simulink model "ThrdRwLtStBkReclnTrgtPosSelc"  (R2018b)
settings: Solver=FixedStepDiscrete  StartTime=0.0  StopTime=10.0  FixedStep=0.01  RelTol=1e-3
undefined symbols (not defined in the file or in its folder): KeSMSw6sAcsEntryThdRwLtStBkReclnUpwdDnwdPos_Val, KeSMSw6sAcsEntryThdRwLtStBkReclnUpwdDnwdPosMax_Val, KeSMSw6sAcsEntryThdRwLtStBkReclnUpwdDnwdPosMin_Val, KeSMSw6sLugThdRwLtStBkReclnUpwdDnwdPos_Val, KeSMSw6sLugThdRwLtStBkReclnUpwdDnwdPosMax_Val, KeSMSw6sLugThdRwLtStBkReclnUpwdDnwdPosMin_Val, KeSMSw6sVIPThdRwLtStBkReclnUpwdDnwdPos_Val, KeSMSw6sVIPThdRwLtStBkReclnUpwdDnwdPosMax_Val, KeSMSw6sVIPThdRwLtStBkReclnUpwdDnwdPosMin_Val, KeSMSwAcsEntryThdRwLtStBkReclnUpwdDnwdPos_Val, KeSMSwAcsEntryThdRwLtStBkReclnUpwdDnwdPosMax_Val, KeSMSwAcsEntryThdRwLtStBkReclnUpwdDnwdPosMin_Val, KeSMSwLugThdRwLtStBkReclnUpwdDnwdPos_Val, KeSMSwLugThdRwLtStBkReclnUpwdDnwdPosMax_Val, KeSMSwLugThdRwLtStBkReclnUpwdDnwdPosMin_Val, KeSMSwVIPThdRwLtStBkReclnUpwdDnwdPos_Val, KeSMSwVIPThdRwLtStBkReclnUpwdDnwdPosMax_Val, KeSMSwVIPThdRwLtStBkReclnUpwdDnwdPosMin_Val
libraries: TrgtPosSelcLib x4
settings Model: Creator=sn2xws  LastModifiedBy=sn2xws
settings DataIOCC: SaveFormat=StructureWithTime
settings OptimizationCC: DefaultParameterBehavior=Inlined  EnhancedBackFolding=on  PassReuseOutputArgsAs=Individual arguments  ZeroExternalMemoryAtStartup=off  ZeroInternalMemoryAtStartup=off  OptimizeBlockOrder=speed  DifferentSizesBufferReuse=on  OptimizationCustomize=off
settings DebuggingCC: ParameterTunabilityLossMsg=error
settings ModelReferenceCC: ModelReferenceNumInstancesAllowed=Single
settings SFSimCC: MATLABDynamicMemAlloc=off
settings RTWCC: SystemTargetFile=autosar.tlc  GenCodeOnly=on  TemplateMakefile=ert_default_tmf  Description=AUTOSAR  GenerateReport=on  IncludeHyperlinkInReport=on  LaunchReport=on  GenerateTraceInfo=on  GenerateTraceReport=on  GenerateTraceReportSl=on  GenerateTraceReportSf=on  GenerateTraceReportEml=on
settings CodeAppCC: ForceParamTrailComments=on  IgnoreCustomStorageClasses=off  OperatorAnnotations=on  SimulinkDataObjDesc=on  SFDataObjDesc=on  InsertBlockDesc=on
settings STFCustomTargetCC: TargetLangStandard=C99 (ISO)  MultiwordLength=256  ParMdlRefBuildCompliant=on  CompOptLevelCompliant=on  IncludeMdlTerminateFcn=off  CombineOutputUpdateFcns=on  SuppressErrorStatus=on  ERTCustomFileBanners=on  SupportNonFinite=off  SupportComplex=off  SupportContinuousTime=off  SupportNonInlinedSFcns=off  RemoveResetFunc=on  MATLABClassNameForMDSCustomization=Simulink.SoftwareTarget.ERTCustomization  AutosarCompliant=on  UseToolchainInfoCompliant=on  LookupTableObjectStructAxisOrder=2,1,3,4,...  LUTObjectStructOrderEvenSpacing=Size,Table,Breakpoints  SystemTargetFile=autosar.tlc
settings ERTTargetCC: TargetLangStandard=C99 (ISO)  ConcurrentExecutionCompliant=off  IncludeMdlTerminateFcn=off  SuppressErrorStatus=on  SupportNonFinite=off  SupportComplex=off  ModelStepFunctionPrototypeControlCompliant=off  CPPClassGenCompliant=off  AutosarCompliant=on  LookupTableObjectStructAxisOrder=2,1,3,4,...  LUTObjectStructOrderEvenSpacing=Size,Table,Breakpoints  InlinedParameterPlacement=NonHierarchical  ERTCustomFileTemplate=example_file_process.tlc

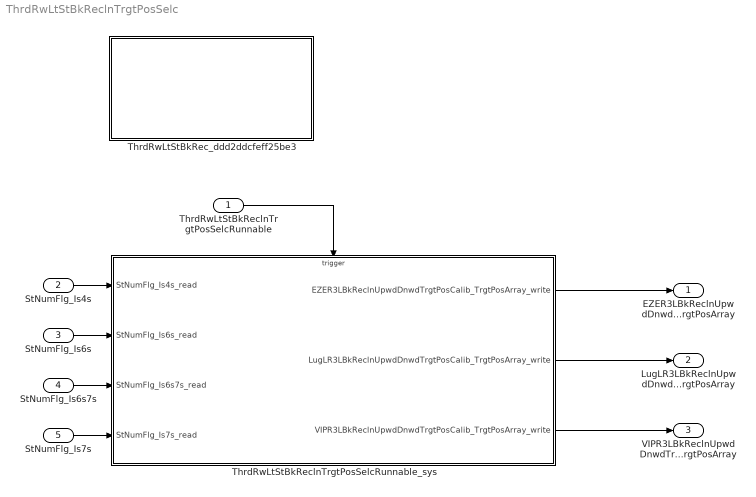
== system ThrdRwLtStBkReclnTrgtPosSelc ==
  ThrdRwLtStBkReclnTrgtPosSelcRunnable : Inport  SampleTime=0.01  OutputFunctionCall=on
  StNumFlg_Is4s : Inport  Port=2  OutDataTypeStr=boolean  PortDimensions=1
  StNumFlg_Is6s : Inport  Port=3  OutDataTypeStr=boolean  PortDimensions=1
  StNumFlg_Is6s7s : Inport  Port=4  OutDataTypeStr=boolean  PortDimensions=1
  StNumFlg_Is7s : Inport  Port=5  OutDataTypeStr=boolean  PortDimensions=1
  ThrdRwLtStBkRec_ddd2ddcfeff25be3 : Subsystem
  ThrdRwLtStBkReclnTrgtPosSelcRunnable_sys : Subsystem
  EZER3LBkReclnUpwdDnwdTrgtPosCalib_TrgtPosArray : Outport  Description=|  OutDataTypeStr=uint16  PortDimensions=3
      | 0:Pos
      | 1:Max
      | 2:Min
  LugLR3LBkReclnUpwdDnwdTrgtPosCalib_TrgtPosArray : Outport  Description=|  Port=2  OutDataTypeStr=uint16  PortDimensions=3
      | 0:Pos
      | 1:Max
      | 2:Min
  VIPR3LBkReclnUpwdDnwdTrgtPosCalib_TrgtPosArray : Outport  Description=|  Port=3  OutDataTypeStr=uint16  PortDimensions=3
      | 0:Pos
      | 1:Max
      | 2:Min
  wires:
  StNumFlg_Is4s/1 -> ThrdRwLtStBkReclnTrgtPosSelcRunnable_sys/1(StNumFlg_Is4s_read)
  StNumFlg_Is6s/1 -> ThrdRwLtStBkReclnTrgtPosSelcRunnable_sys/2(StNumFlg_Is6s_read)
  StNumFlg_Is6s7s/1 -> ThrdRwLtStBkReclnTrgtPosSelcRunnable_sys/3(StNumFlg_Is6s7s_read)
  StNumFlg_Is7s/1 -> ThrdRwLtStBkReclnTrgtPosSelcRunnable_sys/4(StNumFlg_Is7s_read)
  ThrdRwLtStBkReclnTrgtPosSelcRunnable_sys/1(EZER3LBkReclnUpwdDnwdTrgtPosCalib_TrgtPosArray_write) -> EZER3LBkReclnUpwdDnwdTrgtPosCalib_TrgtPosArray/1
  ThrdRwLtStBkReclnTrgtPosSelcRunnable_sys/2(LugLR3LBkReclnUpwdDnwdTrgtPosCalib_TrgtPosArray_write) -> LugLR3LBkReclnUpwdDnwdTrgtPosCalib_TrgtPosArray/1
  ThrdRwLtStBkReclnTrgtPosSelcRunnable_sys/3(VIPR3LBkReclnUpwdDnwdTrgtPosCalib_TrgtPosArray_write) -> VIPR3LBkReclnUpwdDnwdTrgtPosCalib_TrgtPosArray/1
  ThrdRwLtStBkReclnTrgtPosSelcRunnable/1 -> ThrdRwLtStBkReclnTrgtPosSelcRunnable_sys/Trigger

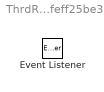
== system ThrdRwLtStBkReclnTrgtPosSelc/ThrdRwLtStBkRec_ddd2ddcfeff25be3 ==
  Event Listener : EventListener  EventName=reset

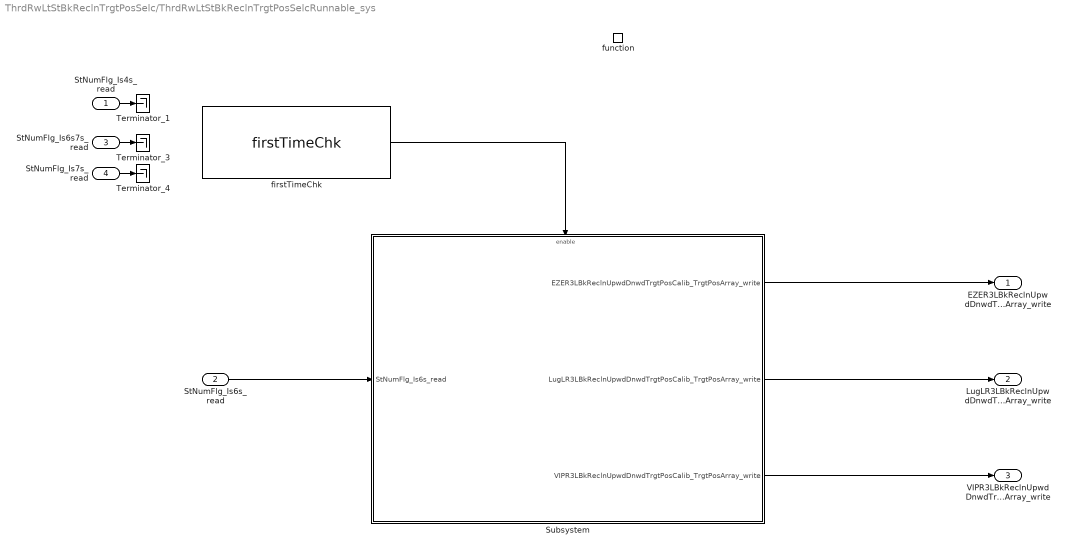
== system ThrdRwLtStBkReclnTrgtPosSelc/ThrdRwLtStBkReclnTrgtPosSelcRunnable_sys ==
  StNumFlg_Is4s_read : Inport
  StNumFlg_Is6s_read : Inport  Port=2
  StNumFlg_Is6s7s_read : Inport  Port=3
  StNumFlg_Is7s_read : Inport  Port=4
  function : TriggerPort  TriggerType=function-call  VariantControl=(inherit)  SampleTimeType=periodic  SampleTime=-1
  Subsystem : Subsystem
  Terminator_1 : Terminator
  Terminator_3 : Terminator
  Terminator_4 : Terminator
  firstTimeChk : TrgtPosSelcLib/firstTimeChk  SystemSampleTime=-1
  EZER3LBkReclnUpwdDnwdTrgtPosCalib_TrgtPosArray_write : Outport
      settings: EnsureOutportIsVirtual=on
  LugLR3LBkReclnUpwdDnwdTrgtPosCalib_TrgtPosArray_write : Outport  Port=2
      settings: EnsureOutportIsVirtual=on
  VIPR3LBkReclnUpwdDnwdTrgtPosCalib_TrgtPosArray_write : Outport  Port=3
      settings: EnsureOutportIsVirtual=on
  wires:
  StNumFlg_Is4s_read/1 -> Terminator_1/1
  StNumFlg_Is6s7s_read/1 -> Terminator_3/1
  StNumFlg_Is7s_read/1 -> Terminator_4/1
  StNumFlg_Is6s_read/1 -> Subsystem/1(StNumFlg_Is6s_read)
  Subsystem/1(EZER3LBkReclnUpwdDnwdTrgtPosCalib_TrgtPosArray_write) -> EZER3LBkReclnUpwdDnwdTrgtPosCalib_TrgtPosArray_write/1
  Subsystem/2(LugLR3LBkReclnUpwdDnwdTrgtPosCalib_TrgtPosArray_write) -> LugLR3LBkReclnUpwdDnwdTrgtPosCalib_TrgtPosArray_write/1
  Subsystem/3(VIPR3LBkReclnUpwdDnwdTrgtPosCalib_TrgtPosArray_write) -> VIPR3LBkReclnUpwdDnwdTrgtPosCalib_TrgtPosArray_write/1
  firstTimeChk/1 -> Subsystem/Enable

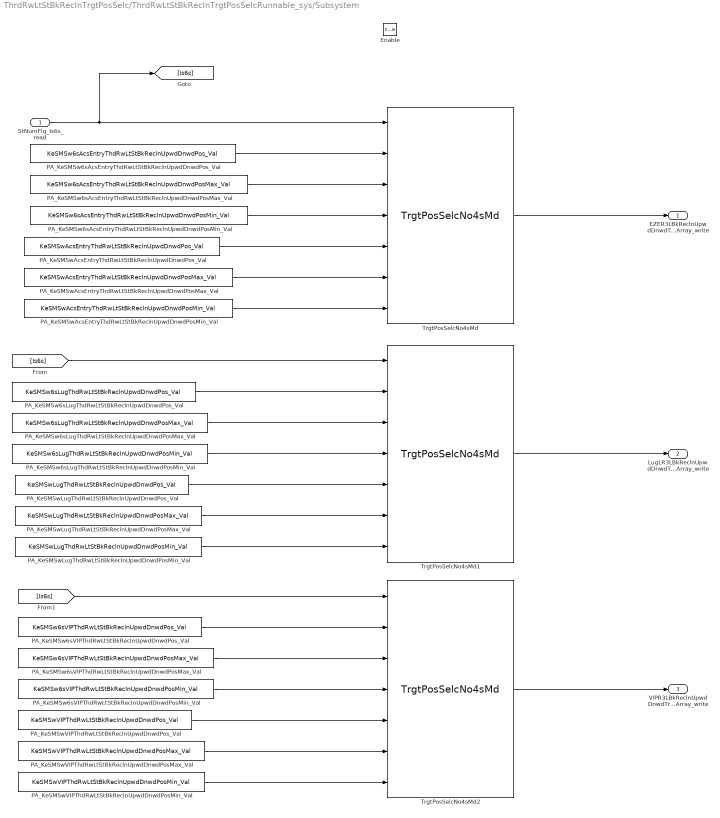
== system ThrdRwLtStBkReclnTrgtPosSelc/ThrdRwLtStBkReclnTrgtPosSelcRunnable_sys/Subsystem ==
  StNumFlg_Is6s_read : Inport
  Enable : EnablePort
  PA_KeSMSw6sAcsEntryThdRwLtStBkReclnUpwdDnwdPosMax_Val : Constant  Value=KeSMSw6sAcsEntryThdRwLtStBkReclnUpwdDnwdPosMax_Val
  PA_KeSMSw6sAcsEntryThdRwLtStBkReclnUpwdDnwdPosMin_Val : Constant  Value=KeSMSw6sAcsEntryThdRwLtStBkReclnUpwdDnwdPosMin_Val
  PA_KeSMSw6sAcsEntryThdRwLtStBkReclnUpwdDnwdPos_Val : Constant  Value=KeSMSw6sAcsEntryThdRwLtStBkReclnUpwdDnwdPos_Val
  PA_KeSMSw6sLugThdRwLtStBkReclnUpwdDnwdPosMax_Val : Constant  Value=KeSMSw6sLugThdRwLtStBkReclnUpwdDnwdPosMax_Val
  PA_KeSMSw6sLugThdRwLtStBkReclnUpwdDnwdPosMin_Val : Constant  Value=KeSMSw6sLugThdRwLtStBkReclnUpwdDnwdPosMin_Val
  PA_KeSMSw6sLugThdRwLtStBkReclnUpwdDnwdPos_Val : Constant  Value=KeSMSw6sLugThdRwLtStBkReclnUpwdDnwdPos_Val
  PA_KeSMSw6sVIPThdRwLtStBkReclnUpwdDnwdPosMax_Val : Constant  Value=KeSMSw6sVIPThdRwLtStBkReclnUpwdDnwdPosMax_Val
  PA_KeSMSw6sVIPThdRwLtStBkReclnUpwdDnwdPosMin_Val : Constant  Value=KeSMSw6sVIPThdRwLtStBkReclnUpwdDnwdPosMin_Val
  PA_KeSMSw6sVIPThdRwLtStBkReclnUpwdDnwdPos_Val : Constant  Value=KeSMSw6sVIPThdRwLtStBkReclnUpwdDnwdPos_Val
  PA_KeSMSwAcsEntryThdRwLtStBkReclnUpwdDnwdPosMax_Val : Constant  Value=KeSMSwAcsEntryThdRwLtStBkReclnUpwdDnwdPosMax_Val
  PA_KeSMSwAcsEntryThdRwLtStBkReclnUpwdDnwdPosMin_Val : Constant  Value=KeSMSwAcsEntryThdRwLtStBkReclnUpwdDnwdPosMin_Val
  PA_KeSMSwAcsEntryThdRwLtStBkReclnUpwdDnwdPos_Val : Constant  Value=KeSMSwAcsEntryThdRwLtStBkReclnUpwdDnwdPos_Val
  PA_KeSMSwLugThdRwLtStBkReclnUpwdDnwdPosMax_Val : Constant  Value=KeSMSwLugThdRwLtStBkReclnUpwdDnwdPosMax_Val
  PA_KeSMSwLugThdRwLtStBkReclnUpwdDnwdPosMin_Val : Constant  Value=KeSMSwLugThdRwLtStBkReclnUpwdDnwdPosMin_Val
  PA_KeSMSwLugThdRwLtStBkReclnUpwdDnwdPos_Val : Constant  Value=KeSMSwLugThdRwLtStBkReclnUpwdDnwdPos_Val
  PA_KeSMSwVIPThdRwLtStBkReclnUpwdDnwdPosMax_Val : Constant  Value=KeSMSwVIPThdRwLtStBkReclnUpwdDnwdPosMax_Val
  PA_KeSMSwVIPThdRwLtStBkReclnUpwdDnwdPosMin_Val : Constant  Value=KeSMSwVIPThdRwLtStBkReclnUpwdDnwdPosMin_Val
  PA_KeSMSwVIPThdRwLtStBkReclnUpwdDnwdPos_Val : Constant  Value=KeSMSwVIPThdRwLtStBkReclnUpwdDnwdPos_Val
  TrgtPosSelcNo4sMd : TrgtPosSelcLib/TrgtPosSelcNo4sMd  SystemSampleTime=-1
  TrgtPosSelcNo4sMd1 : TrgtPosSelcLib/TrgtPosSelcNo4sMd  SystemSampleTime=-1
  TrgtPosSelcNo4sMd2 : TrgtPosSelcLib/TrgtPosSelcNo4sMd  SystemSampleTime=-1
  EZER3LBkReclnUpwdDnwdTrgtPosCalib_TrgtPosArray_write : Outport
      settings: EnsureOutportIsVirtual=on
  LugLR3LBkReclnUpwdDnwdTrgtPosCalib_TrgtPosArray_write : Outport  Port=2
      settings: EnsureOutportIsVirtual=on
  VIPR3LBkReclnUpwdDnwdTrgtPosCalib_TrgtPosArray_write : Outport  Port=3
      settings: EnsureOutportIsVirtual=on
  wires:
  StNumFlg_Is6s_read/1 -> [Is6s], TrgtPosSelcNo4sMd/1
  TrgtPosSelcNo4sMd1/1 -> LugLR3LBkReclnUpwdDnwdTrgtPosCalib_TrgtPosArray_write/1
  TrgtPosSelcNo4sMd2/1 -> VIPR3LBkReclnUpwdDnwdTrgtPosCalib_TrgtPosArray_write/1
  TrgtPosSelcNo4sMd/1 -> EZER3LBkReclnUpwdDnwdTrgtPosCalib_TrgtPosArray_write/1
  [Is6s] -> TrgtPosSelcNo4sMd1/1
  PA_KeSMSw6sAcsEntryThdRwLtStBkReclnUpwdDnwdPosMax_Val/1 -> TrgtPosSelcNo4sMd/3
  PA_KeSMSw6sAcsEntryThdRwLtStBkReclnUpwdDnwdPosMin_Val/1 -> TrgtPosSelcNo4sMd/4
  PA_KeSMSw6sAcsEntryThdRwLtStBkReclnUpwdDnwdPos_Val/1 -> TrgtPosSelcNo4sMd/2
  PA_KeSMSw6sLugThdRwLtStBkReclnUpwdDnwdPosMax_Val/1 -> TrgtPosSelcNo4sMd1/3
  PA_KeSMSw6sLugThdRwLtStBkReclnUpwdDnwdPos_Val/1 -> TrgtPosSelcNo4sMd1/2
  PA_KeSMSw6sLugThdRwLtStBkReclnUpwdDnwdPosMin_Val/1 -> TrgtPosSelcNo4sMd1/4
  [Is6s] -> TrgtPosSelcNo4sMd2/1
  PA_KeSMSw6sVIPThdRwLtStBkReclnUpwdDnwdPosMax_Val/1 -> TrgtPosSelcNo4sMd2/3
  PA_KeSMSw6sVIPThdRwLtStBkReclnUpwdDnwdPos_Val/1 -> TrgtPosSelcNo4sMd2/2
  PA_KeSMSw6sVIPThdRwLtStBkReclnUpwdDnwdPosMin_Val/1 -> TrgtPosSelcNo4sMd2/4
  PA_KeSMSwAcsEntryThdRwLtStBkReclnUpwdDnwdPosMax_Val/1 -> TrgtPosSelcNo4sMd/6
  PA_KeSMSwAcsEntryThdRwLtStBkReclnUpwdDnwdPosMin_Val/1 -> TrgtPosSelcNo4sMd/7
  PA_KeSMSwAcsEntryThdRwLtStBkReclnUpwdDnwdPos_Val/1 -> TrgtPosSelcNo4sMd/5
  PA_KeSMSwLugThdRwLtStBkReclnUpwdDnwdPosMax_Val/1 -> TrgtPosSelcNo4sMd1/6
  PA_KeSMSwLugThdRwLtStBkReclnUpwdDnwdPosMin_Val/1 -> TrgtPosSelcNo4sMd1/7
  PA_KeSMSwLugThdRwLtStBkReclnUpwdDnwdPos_Val/1 -> TrgtPosSelcNo4sMd1/5
  PA_KeSMSwVIPThdRwLtStBkReclnUpwdDnwdPosMax_Val/1 -> TrgtPosSelcNo4sMd2/6
  PA_KeSMSwVIPThdRwLtStBkReclnUpwdDnwdPos_Val/1 -> TrgtPosSelcNo4sMd2/5
  PA_KeSMSwVIPThdRwLtStBkReclnUpwdDnwdPosMin_Val/1 -> TrgtPosSelcNo4sMd2/7
